simulink model "sistema"  (R2026a)
settings: Solver=VariableStepAuto
settings DataIOCC: TimeSaveName=t
settings DebuggingCC: ArtificialAlgebraicLoopMsg=none  MaxConsecutiveZCsMsg=none

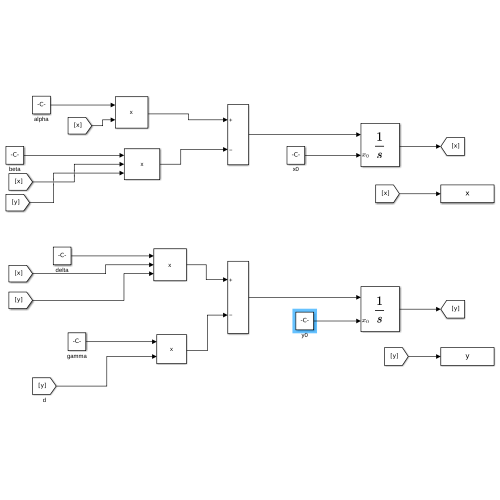
[thumbnail: Simulink's stored preview of the top-level diagram]
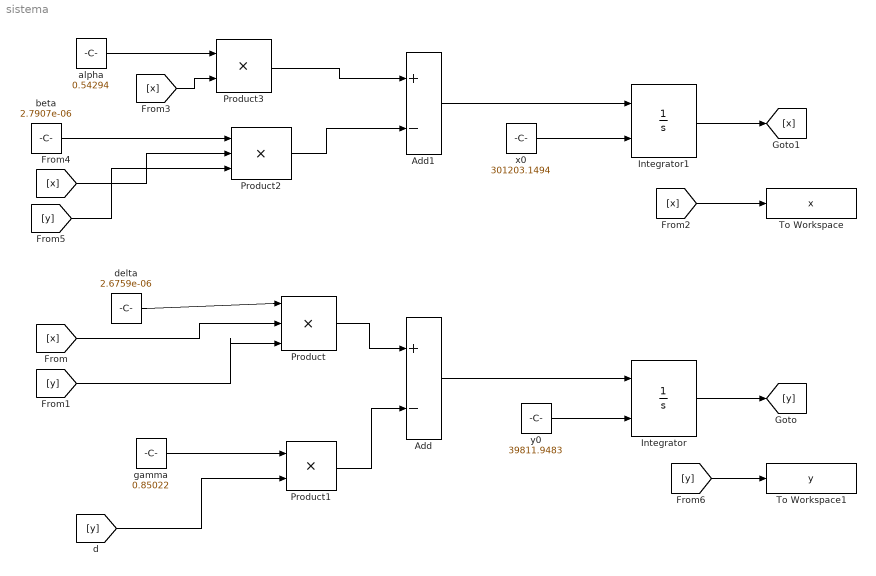
== system sistema ==
  Add : Sum  Inputs=+-
  Add1 : Sum  Inputs=+-
  Integrator : Integrator  InitialConditionSource=external
  Integrator1 : Integrator  InitialConditionSource=external
  Product : Product  Inputs=3
  Product1 : Product
  Product2 : Product  Inputs=3
  Product3 : Product
  To Workspace : ToWorkspace  VariableName=x  SampleTime=-1
  To Workspace1 : ToWorkspace  VariableName=y  SampleTime=-1
  alpha : Constant  Value=0.54294
  beta : Constant  Value=2.7907e-06
  delta : Constant  Value=2.6759e-06
  gamma : Constant  Value=0.85022
  x0 : Constant  Value=301203.1494
  y0 : Constant  Value=39811.9483
  wires:
  Product/1 -> Add/1
  Add/1 -> Integrator/1
  Product1/1 -> Add/2
  y0/1 -> Integrator/2
  Integrator/1 -> [y]
  gamma/1 -> Product1/1
  [y] -> Product1/2
  delta/1 -> Product/1
  [x] -> Product/2
  [y] -> Product/3
  x0/1 -> Integrator1/2
  Add1/1 -> Integrator1/1
  Integrator1/1 -> [x]
  [x] -> Product3/2
  Product3/1 -> Add1/1
  Product2/1 -> Add1/2
  alpha/1 -> Product3/1
  beta/1 -> Product2/1
  [x] -> Product2/2
  [y] -> Product2/3
  [x] -> To Workspace/1
  [y] -> To Workspace1/1
